simulink model "lab4_simulink"  (R2023b)
settings: Solver=FixedStepAuto  StartTime=0.0  StopTime=5  FixedStep=0.001  RelTol=1e-3
values from neighbouring files (symbols this model uses):
  bias = 1    [matlab_data.m]
  phase = 1    [matlab_data.m]
undefined symbols (not defined in the file or in its folder): amplitude, frequency
libraries: instrumentseriallib x3
settings Model: Creator=dinhn  LastModifiedBy=deniskirbaba
settings OptimizationCC: ReuseModelBlockBuffer=off
settings HardwareCC: ProdBitPerPointer=32  ProdBitPerSizeT=32  ProdBitPerPtrDiffT=32  ProdLargestAtomicInteger=Long  ProdLargestAtomicFloat=Double  ProdWordSize=32  ProdHWDeviceType=ARM Compatible->ARM Cortex-M

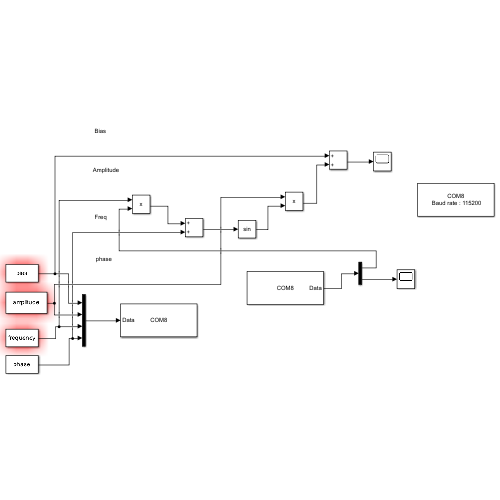
[thumbnail: Simulink's stored preview of the top-level diagram]
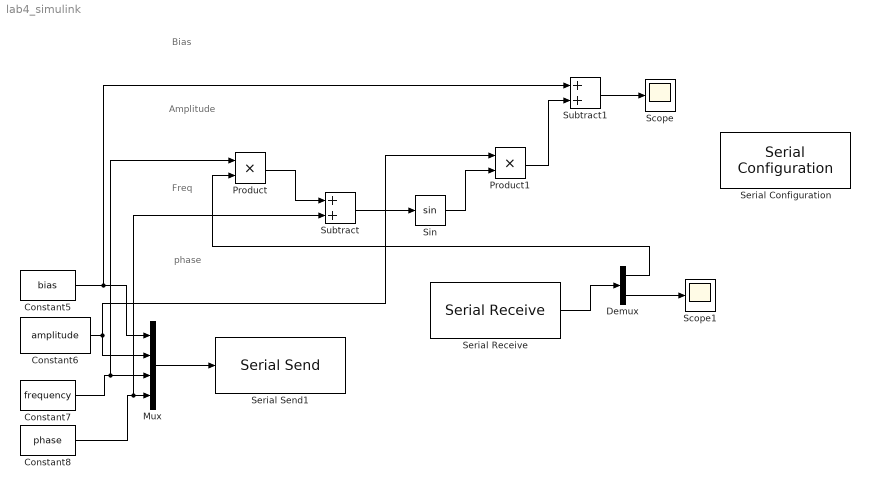
== system lab4_simulink ==
  note: phase
  note: Freq
  note: Amplitude
  note: Bias
  Constant5 : Constant  Value=bias
  Constant6 : Constant  Value=amplitude
  Constant7 : Constant  Value=frequency
  Constant8 : Constant  Value=phase
  Demux : Demux  Outputs=2
  Mux : Mux
  Product : Product
  Product1 : Product
  Scope : Scope
  Scope1 : Scope
  Serial Configuration : instrumentseriallib/Serial Configuration  Priority=-200000  PortSel=COM8  Port=COM8  ComPort=COM8  BaudRate=115200  DataBits=8  Parity=none  StopBits=1  ByteOrder=little-endian  FlowControl=none  Timeout=0.01  SimulateUsing=Interpreted execution  BlockInModel=on  aMode=1
  Serial Receive : instrumentseriallib/Serial Receive  Priority=1  PortSel=COM8  Port=COM8  ComPort=COM8  DataType=single  SaveDataType=uint8  ToggleHeader=on  Header='NNNN'  ToggleTerminator=on  Terminator=Custom terminator  CustomTerminator='EEEE'  InputFormat=Column major  ToggleDataSize=on  DataSize=[2 1]  EnableBlockingMode=on  ActionDataUnavailable=Output last received value  ActionWhenDataUnavailable=Output last received value  CustomValue=0  SampleTime=0.01  SimulateUsing=Interpreted execution  BlockInModel=on  aMode=1
  Serial Send1 : instrumentseriallib/Serial Send  Priority=1  PortSel=COM8  Port=COM8  ComPort=COM8  Header='NNNN'  Terminator=Custom terminator  CustomTerminator='EEEE'  EnableBlockingMode=on  SimulateUsing=Interpreted execution  BlockInModel=on  aMode=1
  Sin : Trigonometry
  Subtract : Sum
  Subtract1 : Sum
  wires:
  Constant7/1 -> Product/1, Mux/3
  Product/1 -> Subtract/1
  Constant8/1 -> Subtract/2, Mux/4
  Subtract/1 -> Sin/1
  Constant6/1 -> Product1/1, Mux/2
  Sin/1 -> Product1/2
  Product1/1 -> Subtract1/2
  Constant5/1 -> Subtract1/1, Mux/1
  Subtract1/1 -> Scope/1
  Mux/1 -> Serial Send1/1
  Serial Receive/1 -> Demux/1
  Demux/2 -> Scope1/1
  Demux/1 -> Product/2
